simulink model "discreteTimeModel"  (R2014b)
settings: Solver=ode4  StartTime=0.0  StopTime=TIME_SIM  FixedStep=STEP_SIZE  RelTol=1e-3
undefined symbols (not defined in the file or in its folder): C, F, G, Gd
settings Model: Creator=Kate  LastModifiedBy=titou
settings DataIOCC: SaveState=on

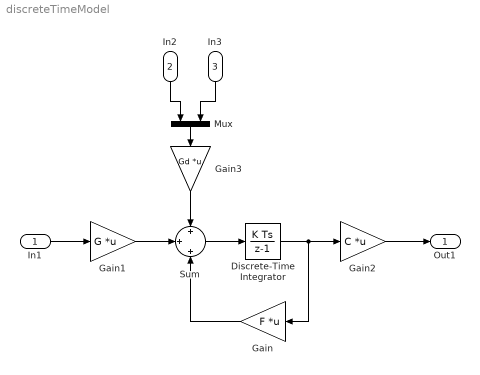
== system discreteTimeModel ==
  In1 : Inport
  In2 : Inport  Port=2
  In3 : Inport  Port=3
  Discrete-Time Integrator : DiscreteIntegrator  InitialConditionSetting=State (most efficient)
  Gain : Gain  Gain=F  Multiplication=Matrix(K*u)
  Gain1 : Gain  Gain=G  Multiplication=Matrix(K*u)
  Gain2 : Gain  Gain=C  Multiplication=Matrix(K*u)
  Gain3 : Gain  Gain=Gd  Multiplication=Matrix(K*u)
  Mux : Mux  Inputs=2
  Sum : Sum  Inputs=+|+|+
  Out1 : Outport
  wires:
  Sum/1 -> Discrete-Time Integrator/1
  Discrete-Time Integrator/1 -> Gain2/1, Gain/1
  Gain/1 -> Sum/3
  Gain1/1 -> Sum/2
  In1/1 -> Gain1/1
  Gain2/1 -> Out1/1
  Gain3/1 -> Sum/1
  Mux/1 -> Gain3/1
  In2/1 -> Mux/1
  In3/1 -> Mux/2
